simulink model "mod3_CIFB_CRFB_3bit"  (Simulink 7.9)
settings: Solver=VariableStepDiscrete  StartTime=0.0  StopTime=simu.trantime  RelTol=1e-3
undefined symbols (not defined in the file or in its folder): a, b, c, Fs, g, mod
libraries: dspsigops x3, dspsrcs4 x1
settings Model: Creator=amyles  LastModifiedBy=Arnaldi Isacco
settings DataIOCC: MaxDataPoints=50000
settings OptimizationCC: InlineParams=on
settings DebuggingCC: UnderspecifiedInitializationDetection=Simplified  InvalidFcnCallConnMsg=none  StrictBusMsg=ErrorOnBusTreatedAsVector
settings ModelReferenceCC: ModelReferenceNumInstancesAllowed=Single
settings CodeAppCC: CustomSymbolStrType=$N$R$M_T
settings GRTTargetCC: CombineOutputUpdateFcns=off  GRTInterface=on

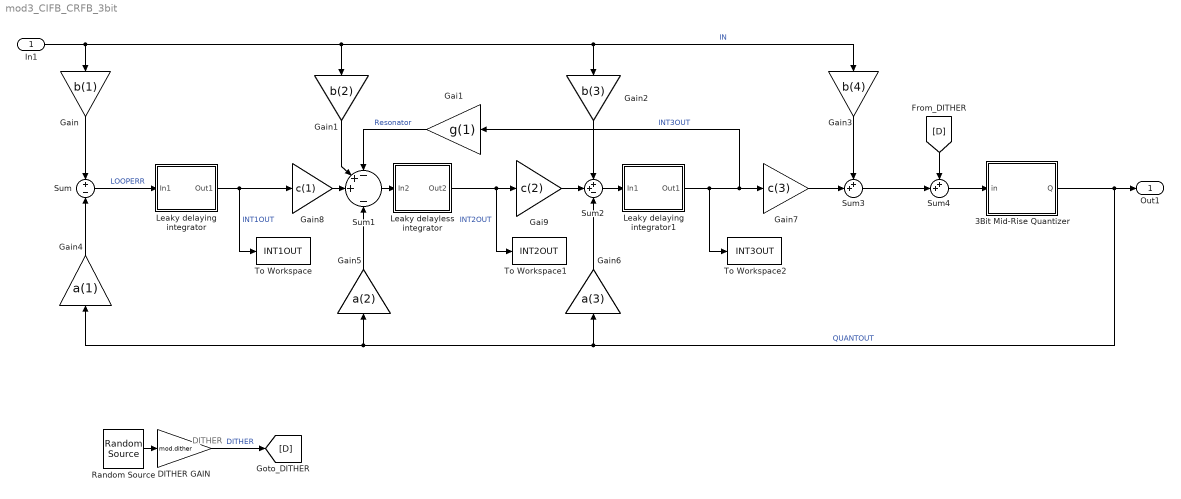
== system mod3_CIFB_CRFB_3bit ==
  note: DITHER
  In1 : Inport
  3Bit Mid-Rise Quantizer : Subsystem
  DITHER GAIN : Gain  Gain=mod.dither  SampleTime=1/Fs
  Gai1 : Gain  Gain=g(1)
  Gai9 : Gain  Gain=c(2)
  Gain : Gain  Gain=b(1)
  Gain1 : Gain  Gain=b(2)
  Gain2 : Gain  Gain=b(3)
  Gain3 : Gain  Gain=b(4)
  Gain4 : Gain  Gain=a(1)
  Gain5 : Gain  Gain=a(2)
  Gain6 : Gain  Gain=a(3)
  Gain7 : Gain  Gain=c(3)
  Gain8 : Gain  Gain=c(1)
  Leaky delaying integrator : Subsystem
  Leaky delaying integrator1 : Subsystem
  Leaky delayless integrator : Subsystem
  Random Source : dspsrcs4/Random Source  SrcType=Uniform  NormMethod=Ziggurat  CltLength=12  MinVal=-1  MaxVal=1  MeanVal=0  VarVal=1  RepMode=Not repeatable  rawSeed=1  IsInherit=off  SampMode=Discrete  SampTime=1/Fs  SampFrame=1  DataType=Double  OutComplex=Real
  Sum : Sum  Inputs=+-  SampleTime=1/Fs
  Sum1 : Sum  Inputs=-++|-  SampleTime=1/Fs
  Sum2 : Sum  Inputs=++-  SampleTime=1/Fs
  Sum3 : Sum  Inputs=++|  SampleTime=1/Fs
  Sum4 : Sum  Inputs=++|
  To Workspace : ToWorkspace  VariableName=INT1OUT  SampleTime=-1
  To Workspace1 : ToWorkspace  VariableName=INT2OUT  SampleTime=-1
  To Workspace2 : ToWorkspace  VariableName=INT3OUT  SampleTime=-1
  Out1 : Outport
  wires:
  In1/1 -> Gain3/1, Gain2/1, Gain1/1, Gain/1  "IN"
  Leaky delaying integrator/1(Out1) -> To Workspace/1, Gain8/1  "INT1OUT"
  Gain8/1 -> Sum1/3
  Leaky delayless integrator/1(Out2) -> To Workspace1/1, Gai9/1  "INT2OUT"
  Gai9/1 -> Sum2/2
  Leaky delaying integrator1/1(Out1) -> Gain7/1, Gai1/1, To Workspace2/1  "INT3OUT"
  Gain7/1 -> Sum3/2
  Gain4/1 -> Sum/2
  Gain/1 -> Sum/1
  Gain1/1 -> Sum1/2
  Gain5/1 -> Sum1/4
  Gai1/1 -> Sum1/1  "Resonator"
  Gain2/1 -> Sum2/1
  Gain6/1 -> Sum2/3
  Gain3/1 -> Sum3/1
  3Bit Mid-Rise Quantizer/1(Q) -> Out1/1, Gain4/1, Gain5/1, Gain6/1  "QUANTOUT"
  Sum/1 -> Leaky delaying integrator/1(In1)  "LOOPERR"
  Sum2/1 -> Leaky delaying integrator1/1(In1)
  Sum1/1 -> Leaky delayless integrator/1(In2)
  Random Source/1 -> DITHER GAIN/1
  DITHER GAIN/1 -> [D]  "DITHER"
  [D] -> Sum4/1
  Sum3/1 -> Sum4/2
  Sum4/1 -> 3Bit Mid-Rise Quantizer/1(in)

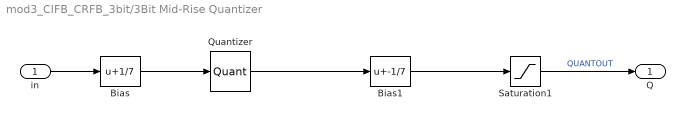
== system mod3_CIFB_CRFB_3bit/3Bit Mid-Rise Quantizer ==
  in : Inport
  Bias : Bias  Bias=1/7
      settings: AttributesFormatString=Need offset to give\nMID-RISE quantiser
  Bias1 : Bias  Bias=-1/7
  Quantizer : Quantizer  QuantizationInterval=2/7  LinearizeAsGain=off  SampleTime=1/Fs
  Saturation1 : Saturate  UpperLimit=mod.qsatout1  LowerLimit=-(mod.qsatout1)
      settings: AttributesFormatString=Limit quantiser\noutput to +/-1
  Q : Outport
  wires:
  Bias/1 -> Quantizer/1
  Quantizer/1 -> Bias1/1
  Bias1/1 -> Saturation1/1
  in/1 -> Bias/1
  Saturation1/1 -> Q/1  "QUANTOUT"

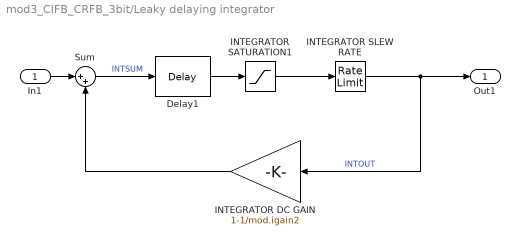
== system mod3_CIFB_CRFB_3bit/Leaky delaying integrator ==
  In1 : Inport
  Delay1 : dspsigops/Delay  InputProcessing=Inherited (this choice will be removed - see release notes)  dly_unit=Samples  delay=1  ic_detail=off  dif_ic_for_ch=off  dif_ic_for_dly=off  ic=0  reset_popup=None
  INTEGRATOR SATURATION1 : Saturate  UpperLimit=mod.isat2  LowerLimit=-(mod.isat2)
  INTEGRATOR SLEW RATE : RateLimiter  RisingSlewLimit=mod.isr1  FallingSlewLimit=-(mod.isr1)  SampleTimeMode=inherited
  INTEGRATOR DC GAIN : Gain  Gain=1-1/mod.igain2
      settings: AttributesFormatString=Integrator leakage\n(model finite integrator dc/LF\ngain in analog modulators)
  Sum : Sum  Inputs=|++
      settings: AttributesFormatString=Integrator summer
  Out1 : Outport
  wires:
  Sum/1 -> Delay1/1  "INTSUM"
  INTEGRATOR DC GAIN/1 -> Sum/2
  INTEGRATOR SATURATION1/1 -> INTEGRATOR SLEW RATE/1
  In1/1 -> Sum/1
  Delay1/1 -> INTEGRATOR SATURATION1/1
  INTEGRATOR SLEW RATE/1 -> Out1/1, INTEGRATOR DC GAIN/1  "INTOUT"

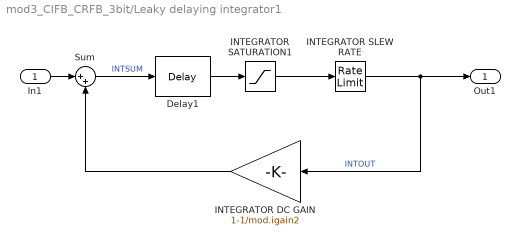
== system mod3_CIFB_CRFB_3bit/Leaky delaying integrator1 ==
  In1 : Inport
  Delay1 : dspsigops/Delay  InputProcessing=Inherited (this choice will be removed - see release notes)  dly_unit=Samples  delay=1  ic_detail=off  dif_ic_for_ch=off  dif_ic_for_dly=off  ic=0  reset_popup=None
  INTEGRATOR SATURATION1 : Saturate  UpperLimit=mod.isat2  LowerLimit=-(mod.isat2)
  INTEGRATOR SLEW RATE : RateLimiter  RisingSlewLimit=mod.isr1  FallingSlewLimit=-(mod.isr1)  SampleTimeMode=inherited
  INTEGRATOR DC GAIN : Gain  Gain=1-1/mod.igain2
      settings: AttributesFormatString=Integrator leakage\n(model finite integrator dc/LF\ngain in analog modulators)
  Sum : Sum  Inputs=|++
      settings: AttributesFormatString=Integrator summer
  Out1 : Outport
  wires:
  Sum/1 -> Delay1/1  "INTSUM"
  INTEGRATOR DC GAIN/1 -> Sum/2
  INTEGRATOR SATURATION1/1 -> INTEGRATOR SLEW RATE/1
  In1/1 -> Sum/1
  Delay1/1 -> INTEGRATOR SATURATION1/1
  INTEGRATOR SLEW RATE/1 -> Out1/1, INTEGRATOR DC GAIN/1  "INTOUT"

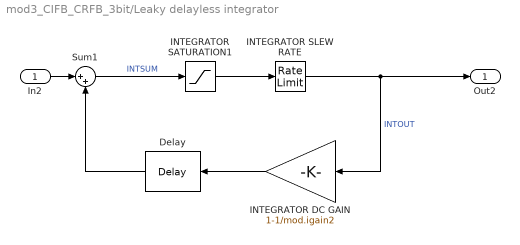
== system mod3_CIFB_CRFB_3bit/Leaky delayless integrator ==
  In2 : Inport
  Delay : dspsigops/Delay  InputProcessing=Inherited (this choice will be removed - see release notes)  dly_unit=Samples  delay=1  ic_detail=off  dif_ic_for_ch=off  dif_ic_for_dly=off  ic=0  reset_popup=None
  INTEGRATOR SATURATION1 : Saturate  UpperLimit=mod.isat2  LowerLimit=-(mod.isat2)
  INTEGRATOR SLEW RATE : RateLimiter  RisingSlewLimit=mod.isr1  FallingSlewLimit=-(mod.isr1)  SampleTimeMode=inherited
  INTEGRATOR DC GAIN : Gain  Gain=1-1/mod.igain2
      settings: AttributesFormatString=Integrator leakage\n(model finite integrator dc/LF\ngain in analog modulators)
  Sum1 : Sum  Inputs=|++
      settings: AttributesFormatString=Integrator summer
  Out2 : Outport
  wires:
  Sum1/1 -> INTEGRATOR SATURATION1/1  "INTSUM"
  INTEGRATOR DC GAIN/1 -> Delay/1
  INTEGRATOR SATURATION1/1 -> INTEGRATOR SLEW RATE/1
  In2/1 -> Sum1/1
  INTEGRATOR SLEW RATE/1 -> Out2/1, INTEGRATOR DC GAIN/1  "INTOUT"
  Delay/1 -> Sum1/2
